simulink model "bdot_sardonyx"  (R2026a)
settings: Solver=VariableStepAuto  StopTime=9000
undefined symbols (not defined in the file): deg, juliandate, rad, s
libraries: vrlib x4, matrix_library x3, aerolibconvert2 x1, aerolibcubesatveh x1, simulink x1, aerolibnav x1
settings Model: Creator=jseon01  LastModifiedBy=jseon01

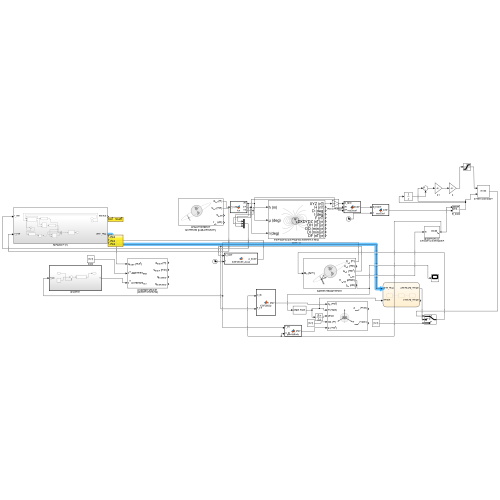
[thumbnail: Simulink's stored preview of the top-level diagram]
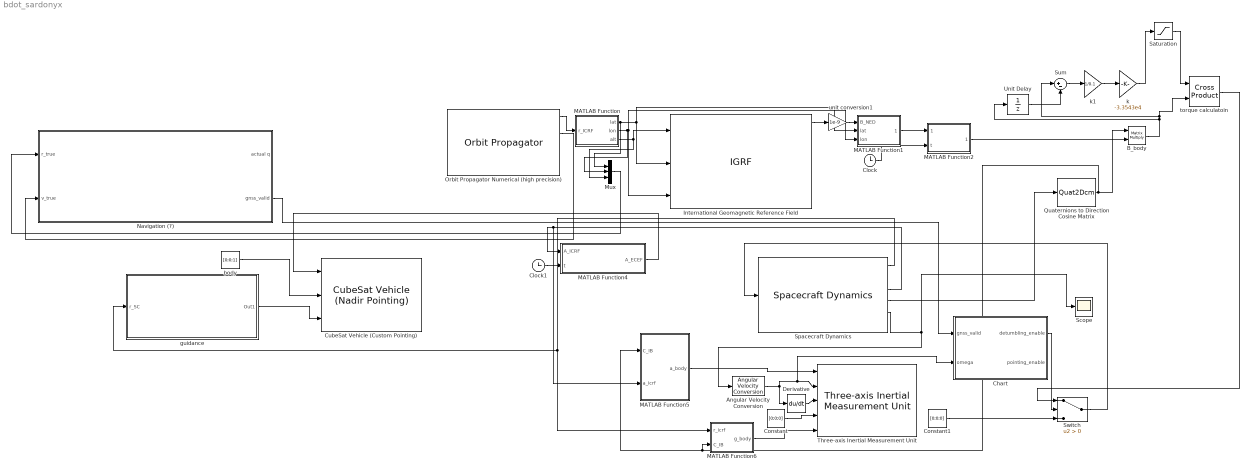
== system bdot_sardonyx ==
  Angular Velocity Conversion : aerolibconvert2/Angular Velocity Conversion  IU=deg/s  OU=rad/s
  B_body : Product  Multiplication=Matrix(*)
  Chart : Stateflow chart  TreatAsAtomicUnit=on
  Clock : Clock
  Clock1 : Clock
  Constant : Constant  Value=[0;0;0]
  Constant1 : Constant  Value=[0;0;0]
  CubeSat Vehicle (Custom Pointing) : aerolibcubesatveh/CubeSat Vehicle (Nadir Pointing)  sim_t0=juliandate(2019, 1, 4, 12, 0, 0)  method=Keplerian Orbital Elements  epoch=juliandate(2000, 1, 1, 12, 0, 0)  a=6978000  ecc=0  incl=97.6  omega=318.55  argp=0  nu=0  truelon=0  arglat=0  lonper=0  r_eci=[0 0 0]  v_eci=[0 0 0]  r_ecef=[0 0 0]  v_ecef=[0 0 0]  lla=[0 0 0]  v_ned=[0 0 0]  euler=[0 0 0]  pqr=[0 0 -0.05168]  pointingMode=Custom Pointing  firstAlignExt=Input port  firstAlign=[0 0 1]  secondAlignExt=Dialog  secondAlign=[0 1 0]  constraintCoord=ECI Axes  firstRefExt=Input port  firstRef=[1 0 0]  secondRefExt=Dialog  secondRef=[0 0 1]  missionRTSource=Dialog  missionRT=6*60*60  missionGS=[38.6270,-90.1994]  missionTOICheck=on  missionTOI=[]  missionEta=55
      settings: LibrarySourceBlock=|
      | aerolibcubesatveh/CubeSat Vehicle
      | (Custom Pointing)
  Derivative : Derivative
  International Geomagnetic Reference Field : IGRF  time_in=off  month=January  day=1
      settings: AttributesFormatString=%<generation>
  MATLAB Function : MATLAB Function  TreatAsAtomicUnit=on
  MATLAB Function1 : MATLAB Function  TreatAsAtomicUnit=on
  MATLAB Function2 : MATLAB Function  TreatAsAtomicUnit=on
  MATLAB Function4 : MATLAB Function  TreatAsAtomicUnit=on
  MATLAB Function5 : MATLAB Function  TreatAsAtomicUnit=on
  MATLAB Function6 : MATLAB Function  TreatAsAtomicUnit=on
  Mux : Mux  Inputs=3
  Navigation (?) : Subsystem
  Orbit Propagator Numerical (high precision) : OrbitPropagator  propagator=Numerical (high precision)  semiMajorAxis=6978000  eccentricity=0  inclination=97.6  raan=318.55  argPeriapsis=86  inertialPosition=[3649700.0 3308200.0 -4676600.0]  inertialVelocity=[-2750.8 6666.4 2573.4]  fixedPosition=[-4142689.0 -2676864.7 -4669861.6]  fixedVelocity=[1452.7 -6720.7 2568.1]  customR=3396200  customMu=4.305e13  customJ2=1.0826269e-03  customOmega=4.06125949e-3  outputTransform=on
  Quaternions to Direction Cosine Matrix : Quat2Dcm
  Saturation : Saturate  UpperLimit=[0.15;0.15;0.15]  LowerLimit=[-0.15;-0.15;-0.15]
  Scope : Scope
      settings: ActiveDisplayYMinimum=-8.7464306228860043  ActiveDisplayYMaximum=8.7987612239477748
  Spacecraft Dynamics : SpacecraftDynamics  forcesIn=off  outputAccel=on  mass=21.137  inertia=[0.229, 0, 0; 0, 0.229, 0; 0, 0, .141]  semiMajorAxis=6978000  eccentricity=0  inclination=97.6  raan=318.55  argPeriapsis=88  attitudeRate=[5;5;5]  gravityModel=Point-mass  useDrag=on  useEphemerisDateRange=off  useThirdBodyGravity=on  sunThirdBodyGravityModel=Oblate ellipsoid (J2)  moonThirdBodyGravityModel=Oblate ellipsoid (J2)  useSRP=on
  Sum : Sum  Inputs=|+-
  Switch : Switch  Criteria=u2 > Threshold  SaturateOnIntegerOverflow=off  InputSameDT=off
  Three-axis Inertial Measurement Unit : aerolibnav/Three-axis Inertial Measurement Unit  units=Metric (MKS)  imu=[0 0 0]  i_Ts=0  dtype_a=on  w_a=190  z_a=0.707  a_sf_cc=[1 0 0; 0 1 0; 0 0 1]  a_bias=[0 0 0]  a_sat="[-inf  -inf  -inf  inf inf inf]"  dtype_g=on  w_g=190  z_g=0.707  g_sf_cc=[1 0 0; 0 1 0; 0 0 1]  g_bias=[0 0 0]  g_sens=[0 0 0]  g_sat="[-inf  -inf  -inf  inf inf inf]"  i_rand=on  i_seeds=[23093 23094 23095 23096 23097 23098]  i_pow=[0.001 0.001 0.001 0.0001 0.0001 0.0001]
  Unit Delay : UnitDelay  InitialCondition=[0;0;0]  SampleTime=0.1
  body : Constant  Value=[0;0;1]
  guidance : Subsystem  TreatAsAtomicUnit=on
  k : Gain  Gain=-3.3543e4
  k1 : Gain  Gain=1/0.1
  torque calculatoin : matrix_library/Cross Product
  unit conversion1 : Gain  Gain=1e-9
  wires:
  International Geomagnetic Reference Field/1 -> unit conversion1/1
  B_body/1 -> torque calculatoin/2, Sum/1, Unit Delay/1
  Quaternions to Direction Cosine Matrix/1 -> MATLAB Function6/2(C_IB), MATLAB Function5/1(C_IB), B_body/1
  MATLAB Function/1(lat) -> Mux/1, MATLAB Function1/2(lat), International Geomagnetic Reference Field/2
  Unit Delay/1 -> Sum/2
  MATLAB Function1/1(B_ECEF) -> MATLAB Function2/1(B_ECEF)
  Clock/1 -> MATLAB Function2/2(t)
  Spacecraft Dynamics/4 -> Quaternions to Direction Cosine Matrix/1
  k/1 -> Saturation/1
  Saturation/1 -> torque calculatoin/1
  Sum/1 -> k1/1
  MATLAB Function/2(lon) -> Mux/2, MATLAB Function1/3(lon), International Geomagnetic Reference Field/3
  unit conversion1/1 -> MATLAB Function1/1(B_NED)
  MATLAB Function2/1(B_ICRF) -> B_body/2
  MATLAB Function/3(alt) -> Mux/3, International Geomagnetic Reference Field/1
  k1/1 -> k/1
  Orbit Propagator Numerical (high precision)/2 -> Navigation (?)/2(v_true)
  Orbit Propagator Numerical (high precision)/1 -> MATLAB Function/1(r_ICRF)
  Mux/1 -> Navigation (?)/1(r_true)
  body/1 -> CubeSat Vehicle (Custom Pointing)/2
  guidance/1(Out1) -> CubeSat Vehicle (Custom Pointing)/3
  Spacecraft Dynamics/3 -> MATLAB Function5/2(a_icrf), MATLAB Function4/1(A_ICRF)
  Clock1/1 -> MATLAB Function4/2(t)
  MATLAB Function4/1(A_ECEF) -> CubeSat Vehicle (Custom Pointing)/1
  Spacecraft Dynamics/5 -> Angular Velocity Conversion/1, Scope/1
  Angular Velocity Conversion/1 -> Derivative/1, Chart/2(omega), Three-axis Inertial Measurement Unit/2
  MATLAB Function5/1(a_body) -> Three-axis Inertial Measurement Unit/1
  Derivative/1 -> Three-axis Inertial Measurement Unit/3
  Spacecraft Dynamics/1 -> MATLAB Function6/1(r_icrf), guidance/1(r_SC)
  Constant/1 -> Three-axis Inertial Measurement Unit/4
  MATLAB Function6/1(g_body) -> Three-axis Inertial Measurement Unit/5
  Switch/1 -> Spacecraft Dynamics/1
  Chart/1(detumbling_enable) -> Switch/2
  torque calculatoin/1 -> Switch/1
  Constant1/1 -> Switch/3
  Navigation (?)/2(gnss_valid) -> Chart/1(gnss_valid)

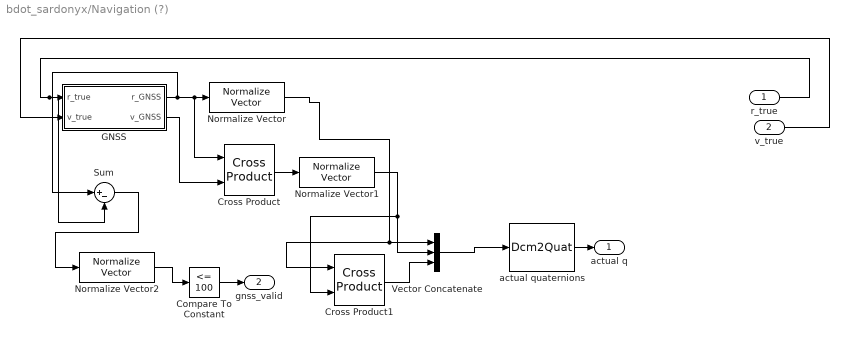
== system bdot_sardonyx/Navigation (?) ==
  r_true : Inport
  v_true : Inport  Port=2
  Compare To Constant : simulink/Logic and Bit Operations/Compare To Constant  relop=<=  const=100  OutDataTypeStr=boolean
  Cross Product : matrix_library/Cross Product
  Cross Product1 : matrix_library/Cross Product
  GNSS : Subsystem  TreatAsAtomicUnit=on
  Normalize Vector : vrlib/Utilities/Normalize Vector  maxzero=0
  Normalize Vector1 : vrlib/Utilities/Normalize Vector  maxzero=0
  Normalize Vector2 : vrlib/Utilities/Normalize Vector  maxzero=0
  Sum : Sum  Inputs=|+-
  Vector Concatenate : Concatenate  NumInputs=3  Mode=Multidimensional array  ConcatenateDimension=2
  actual quaternions : Dcm2Quat
  actual q : Outport
  gnss_valid : Outport  Port=2
  wires:
  actual quaternions/1 -> actual q/1
  Normalize Vector/1 -> Cross Product1/1, Vector Concatenate/1
  GNSS/2(v_GNSS) -> Cross Product/2
  Cross Product/1 -> Normalize Vector1/1
  v_true/1 -> GNSS/2(v_true)
  r_true/1 -> Sum/2, GNSS/1(r_true)
  Normalize Vector1/1 -> Cross Product1/2, Vector Concatenate/2
  GNSS/1(r_GNSS) -> Sum/1, Cross Product/1, Normalize Vector/1
  Cross Product1/1 -> Vector Concatenate/3
  Vector Concatenate/1 -> actual quaternions/1
  Sum/1 -> Normalize Vector2/1
  Normalize Vector2/1 -> Compare To Constant/1
  Compare To Constant/1 -> gnss_valid/1

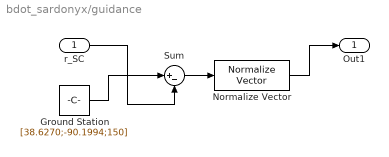
== system bdot_sardonyx/guidance ==
  r_SC : Inport
  Ground Station : Constant  Value=[38.6270;-90.1994;150]
  Normalize Vector : vrlib/Utilities/Normalize Vector  maxzero=0
  Sum : Sum  Inputs=|+-
  Out1 : Outport
  wires:
  r_SC/1 -> Sum/2
  Ground Station/1 -> Sum/1
  Sum/1 -> Normalize Vector/1
  Normalize Vector/1 -> Out1/1

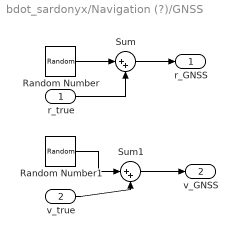
== system bdot_sardonyx/Navigation (?)/GNSS ==
  r_true : Inport
  v_true : Inport  Port=2
  Random Number : RandomNumber  Variance=25  SampleTime=0.1
  Random Number1 : RandomNumber  Variance=0.01  SampleTime=0.1
  Sum : Sum  Inputs=|++
  Sum1 : Sum  Inputs=|++
  r_GNSS : Outport
  v_GNSS : Outport  Port=2
  wires:
  Sum/1 -> r_GNSS/1
  r_true/1 -> Sum/2
  Random Number/1 -> Sum/1
  Random Number1/1 -> Sum1/1
  v_true/1 -> Sum1/2
  Sum1/1 -> v_GNSS/1

== stateflow chart bdot_sardonyx/Chart ==
  state Detumble
    entry:
    detumbling_enable=true;
    pointing_enable=false;
  state Navigation
    entry:
    detumbling_enable=false;
    pointing_enable=false;
  state Pointing
    entry:
    detumbling_enable=false;
    pointing_enable=true;
  (default) -> Detumble
  Detumble -> Navigation : [abs(omega) < 0.05]
  Navigation -> Pointing : [gnss_valid == 1]
  data: detumbling_enable output boolean size=1 =0; gnss_valid input; omega input; pointing_enable output

== matlab function bdot_sardonyx/MATLAB Function1 ==
  data: B_NED input; B_ECEF output; lat input; lon input
function B_ECEF = ned2ecef(B_NED, lat, lon)

phi = deg2rad(lat);
lambda = deg2rad(lon);

C = [
    -sin(phi)*cos(lambda), -sin(lambda), -cos(phi)*cos(lambda);
    -sin(phi)*sin(lambda),  cos(lambda), -cos(phi)*sin(lambda);
     cos(phi),             0,            -sin(phi)
    ];

B_ECEF = C * B_NED;

end

== matlab function bdot_sardonyx/MATLAB Function ==
  data: r_ICRF input; lat output; lon output; alt output
function [lat,lon,alt] = fcn(r_ICRF)

x = r_ICRF(1);
y = r_ICRF(2);
z = r_ICRF(3);

Re = 6378.137e3;

r = sqrt(x^2+y^2+z^2);

lat = asin(z/r);
lon = atan2(y,x);

lat = rad2deg(lat);
lon = rad2deg(lon);

alt = r-Re;

end

== matlab function bdot_sardonyx/MATLAB Function2 ==
  data: B_ECEF input; B_ICRF output; t input
function B_ICRF = ecef2icrf(B_ECEF, t)

% Earth rotation rate [rad/s]
omega_E = 7.2921151467e-5;

% initial angle (simplified)
theta0 = 0;

% Earth rotation angle
theta = theta0 + omega_E*t;

% Rotation matrix
C = [
    cos(theta) -sin(theta) 0;
    sin(theta)  cos(theta) 0;
    0           0          1
];

% Convert
B_ICRF = C * B_ECEF;

end

== matlab function bdot_sardonyx/MATLAB Function4 ==
  data: A_ICRF input; A_ECEF output; t input
function A_ECEF = ICRF2ECEF_Accel(A_ICRF, t)
%#codegen
% Convert acceleration vector from ICRF (ECI) to ECEF
%
% Inputs:
%   A_ICRF : 3x1 acceleration vector [m/s^2]
%   t      : simulation time [s]
%
% Output:
%   A_ECEF : 3x1 acceleration vector [m/s^2]

% Earth rotation rate (rad/s)
omegaEarth = 7.2921159e-5;

% Earth rotation angle
theta = omegaEarth * t;

% ECI -> ECEF rotation matrix
R = [ cos(theta),  sin(theta), 0;
     -sin(theta),  cos(theta), 0;
      0,           0,          1];

A_ECEF = R * A_ICRF;

== matlab function bdot_sardonyx/MATLAB Function5 ==
  data: C_IB input; a_body output; a_icrf input
function a_body = ICRF2Body(C_IB, a_icrf)
% C_IB = Direction Cosine Matrix from ICRF to Body

a_body = C_IB * a_icrf;
end

== matlab function bdot_sardonyx/MATLAB Function6 ==
  data: r_icrf input; g_body output; C_IB input
function g_body = gravityBody(r_icrf, C_IB)

mu = 3.986004418e14;

r = norm(r_icrf);

g_icrf = -mu/r^3 * r_icrf;

g_body = C_IB * g_icrf;

end
